simulink model "peredatcha"  (Simulink 8.7)
settings: Solver=VariableStepAuto  SolverMode=SingleTasking  StartTime=0.0  StopTime=250  FixedStep=1  RelTol=1e-3  AbsTol=1e6
libraries: KP x6, commblksprivate x2, dspsrcs4 x1
settings Model: Creator=KDFX Team  LastModifiedBy=KDFX Team
settings DataIOCC: SignalLoggingSaveFormat=ModelDataLogs  SignalLoggingName=sigsOut
settings OptimizationCC: BooleanDataType=off
settings DebuggingCC: SaveWithParameterizedLinksMsg=none  SignalResolutionControl=TryResolveAllWithWarning  MultiTaskDSMMsg=warning  MultiTaskCondExecSysMsg=none
settings HardwareCC: TargetUnknown=on
settings GRTTargetCC: GeneratePreprocessorConditionals=Use local settings  CombineOutputUpdateFcns=off  GRTInterface=on

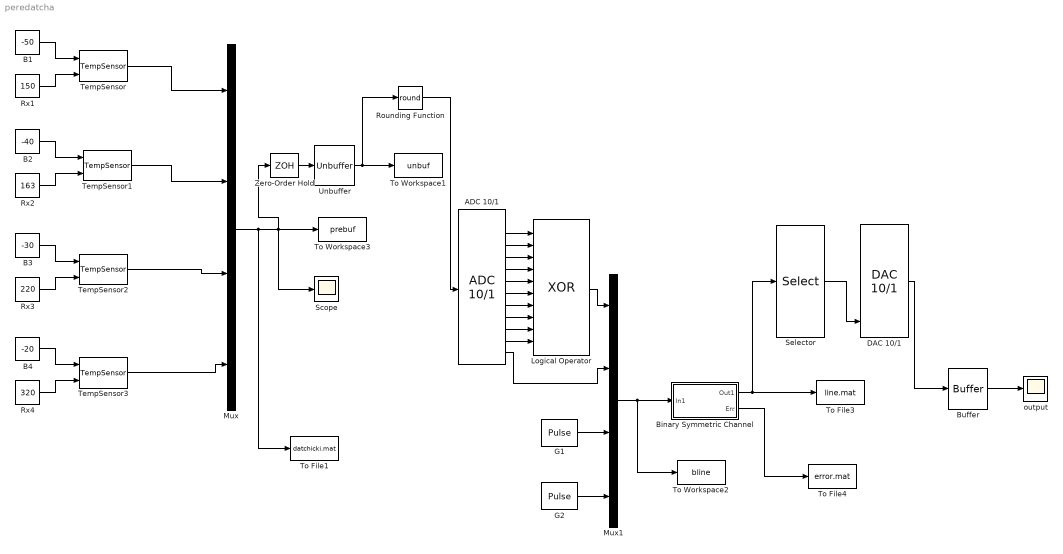
== system peredatcha ==
  ADC 10/1 : KP/ADC 10//1
  B1 : Constant  Value=-50  SampleTime=0
  B2 : Constant  Value=-40  SampleTime=0
  B3 : Constant  Value=-30  SampleTime=0
  B4 : Constant  Value=-20  SampleTime=0
  Binary Symmetric Channel : Subsystem  AncestorBlock=commchan2/Binary Symmetric Channel  mask(Binary Symmetric Channel){P=0.000000, s=2137, E=on}
      mask prompts: P "Error probability:"; s "Initial seed:"; E "Output error vector"
      mask help:
      | Add binary errors to the input signal. The error probability can be a scalar or a vector with the same length as the input vector length.
      |
      | The optional second output is the error vector.
      mask init:
      | commblkbschan(P,s)
      mask Help: helpview(commbhelp)
      mask Display:
      | plot(0,0,100,100,[05 15 10 10 05 10 18 14 13 7.5 13 41 44 47 50 53 57 59 100-[13 7.5 13 14 18 10 5 10 10 15 5]],[70 70 70 85 92 85 79 82 90 88.5 90 90 87 93 87 93 87 90 90 88.5 90 82 79 85 92 85 70 70 70]);
      | disp('BSC')
  Buffer : Buffer  N=4  TreatMby1Signals=One channel  OutputFrames=off
  DAC 10/1 : KP/DAC 10//1
  G1 : DiscretePulseGenerator  PhaseDelay=1
  G2 : DiscretePulseGenerator  Period=4  PulseWidth=2  PhaseDelay=2
  Logical Operator : Logic  Operator=XOR  Inputs=10
  Mux : Mux
  Mux1 : Mux
  Rounding Function : Rounding  Operator=round
  Rx1 : Constant  Value=150  SampleTime=0
  Rx2 : Constant  Value=163  SampleTime=0
  Rx3 : Constant  Value=220  SampleTime=0
  Rx4 : Constant  Value=320  SampleTime=0
  Scope : Scope
  Selector : Selector  InputPortWidth=13  IndexOptions=Index vector (dialog)  Indices=[1 2 3 4 5 6 7 8 9 10]  OutputSizes=1
  TempSensor : KP/TempSensor
  TempSensor1 : KP/TempSensor
      link override Gain: Gain=0.813
  TempSensor2 : KP/TempSensor
      link override Gain: Gain=0.807
  TempSensor3 : KP/TempSensor
      link override Gain: Gain=0.835
  To File1 : ToFile  Filename=datchicki.mat  MatrixName=datchiki
  To File3 : ToFile  Filename=line.mat  MatrixName=line
  To File4 : ToFile  Filename=error.mat  MatrixName=error
  To Workspace1 : ToWorkspace  VariableName=unbuf  SampleTime=-1
  To Workspace2 : ToWorkspace  VariableName=bline  SampleTime=-1
  To Workspace3 : ToWorkspace  VariableName=prebuf  SampleTime=-1
  Unbuffer : Unbuffer  ic=4  SampleBasedProcessing=Same as frame based
  Zero-Order Hold : ZeroOrderHold
  output : Scope
  wires:
  B1/1 -> TempSensor/1
  Rx1/1 -> TempSensor/2
  B2/1 -> TempSensor1/1
  Rx2/1 -> TempSensor1/2
  B3/1 -> TempSensor2/1
  Rx3/1 -> TempSensor2/2
  B4/1 -> TempSensor3/1
  Rx4/1 -> TempSensor3/2
  TempSensor3/1 -> Mux/4
  Mux/1 -> To Workspace3/1, Zero-Order Hold/1, Scope/1, To File1/1
  Rounding Function/1 -> ADC 10/1/1
  Logical Operator/1 -> Mux1/1
  G1/1 -> Mux1/3
  G2/1 -> Mux1/4
  Mux1/1 -> Binary Symmetric Channel/1(In1), To Workspace2/1
  Binary Symmetric Channel/1(Out1) -> To File3/1, Selector/1
  Binary Symmetric Channel/2(Err) -> To File4/1
  Selector/1 -> DAC 10/1/11
  DAC 10/1/1 -> Buffer/1
  Buffer/1 -> output/1
  ADC 10/1/12 -> Mux1/2
  TempSensor/1 -> Mux/1
  TempSensor1/1 -> Mux/2
  TempSensor2/1 -> Mux/3
  Unbuffer/1 -> To Workspace1/1, Rounding Function/1
  Zero-Order Hold/1 -> Unbuffer/1
  ADC 10/1/11 -> Logical Operator/10
  ADC 10/1/10 -> Logical Operator/9
  ADC 10/1/9 -> Logical Operator/8
  ADC 10/1/8 -> Logical Operator/7
  ADC 10/1/7 -> Logical Operator/6
  ADC 10/1/6 -> Logical Operator/5
  ADC 10/1/5 -> Logical Operator/4
  ADC 10/1/4 -> Logical Operator/3
  ADC 10/1/3 -> Logical Operator/2
  ADC 10/1/2 -> Logical Operator/1

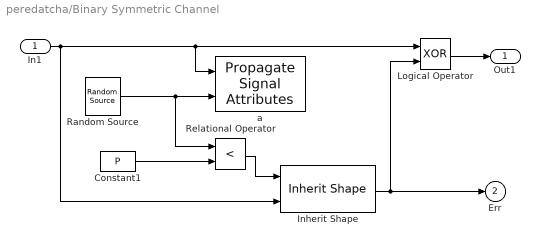
== system peredatcha/Binary Symmetric Channel ==
  In1 : Inport
  Constant1 : Constant  Value=P
  Inherit Shape : commblksprivate/Inherit Shape
  Logical Operator : Logic  Operator=XOR  OutDataTypeStr=float('double')
  Random Source : dspsrcs4/Random Source  SrcType=Uniform  NormMethod=Ziggurat  CltLength=12  MinVal=0  MaxVal=1  MeanVal=0  VarVal=1  RepMode=Specify seed  rawSeed=s  IsInherit=on  SampMode=Discrete  SampTime=1  SampFrame=1  DataType=Double  OutComplex=Real  OutputFrames=on
  Relational Operator : RelationalOperator  Operator=<  OutDataTypeStr=float('double')  InputSameDT=on
  a : commblksprivate/Propagate Signal Attributes
  Out1 : Outport
  Err : Outport  Port=2
  wires:
  Random Source/1 -> a/2, Relational Operator/1
  Constant1/1 -> Relational Operator/2
  In1/1 -> a/1, Logical Operator/1, Inherit Shape/2
  Logical Operator/1 -> Out1/1
  Inherit Shape/1 -> Logical Operator/2, Err/1
  Relational Operator/1 -> Inherit Shape/1
